simulink model "Mechanik_FensterSchlitten"  (R2021a)
settings: Solver=ode23s  StartTime=0.0  StopTime=10  MaxStep=1e-3  MinStep=1e-5  RelTol=1e-5  AbsTol=1e-5
values from neighbouring files (symbols this model uses):
  c = 10000    [Konstanten.m]
  d = 50    [Konstanten.m]
  da = 0.022    [Konstanten.m]
  eta = 0.7    [Konstanten.m]
  FR_Gleit = 4*mueG*FD    (= 27.5555)    [Konstanten.m]
  FR_Haft = (mF+mS)*g+0.1    (= 31.492)    [Konstanten.m]
  g = 9.81    [Konstanten.m]
  i = 1/49    (= 0.0204081632653)    [Konstanten.m]
  J = 1.8    [Konstanten.m]
  k3 = k4    (= 0.0315)    [Konstanten.m]
  k4 = M_Mot/Ia    (= 0.0315)    [Konstanten.m]
  ki = 100    [Konstanten.m]
  ki_U = 100    [Konstanten.m]
  kp = 100    [Konstanten.m]
  kp_U = 100    [Konstanten.m]
  L = Ta*Ra    (= 0.00161202272727)    [Konstanten.m]
  mF = 2.3    [Konstanten.m]
  mS = 0.9    [Konstanten.m]
  Ra = (Ua-UbN)/Ia    (= 1.81534090909)    [Konstanten.m]
settings Model: Creator=johannes  LastModifiedBy=johannes
settings SolverCC: ZeroCrossAlgorithm=Adaptive
settings DebuggingCC: IgnoredZcDiagnostic=none

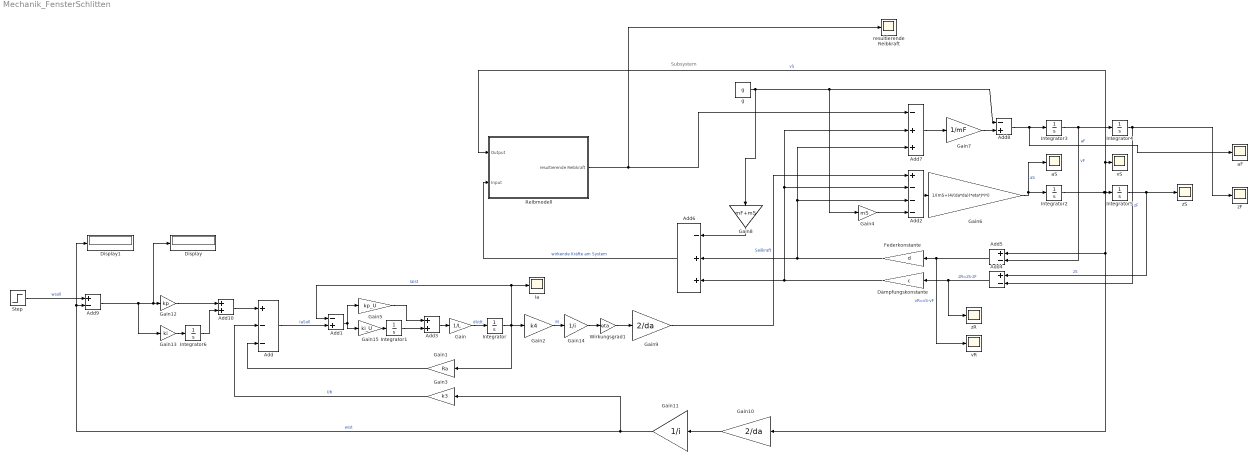
== system Mechanik_FensterSchlitten ==
  note: Subsystem
  Add : Sum  Inputs=+--
  Add1 : Sum  Inputs=-+
  Add10 : Sum
  Add2 : Sum  Inputs=+---
  Add3 : Sum
  Add4 : Sum  Inputs=+-
  Add5 : Sum  Inputs=+-
  Add6 : Sum  Inputs=-++
  Add7 : Sum  Inputs=-++
  Add8 : Sum  Inputs=-+
  Add9 : Sum  Inputs=+-
  Display : Display
  Display1 : Display
  Dämpfungskonstante : Gain  Gain=c
  Federkonstante : Gain  Gain=d
  Gain : Gain  Gain=1/L
  Gain1 : Gain  Gain=Ra
  Gain10 : Gain  Gain=2/da
  Gain11 : Gain  Gain=1/i
  Gain12 : Gain  Gain=kp
  Gain13 : Gain  Gain=ki
  Gain14 : Gain  Gain=1/i
  Gain15 : Gain  Gain=ki_U
  Gain2 : Gain  Gain=k4
  Gain3 : Gain  Gain=k3
  Gain4 : Gain  Gain=mS
  Gain5 : Gain  Gain=kp_U
  Gain6 : Gain  Gain=1/(mS+(4/(da*da))*eta*J*i*i)
  Gain7 : Gain  Gain=1/mF
  Gain8 : Gain  Gain=mF+mS
  Gain9 : Gain  Gain=2/da
  Ia : Scope
  Integrator{,1,3..6} (6 alike) : Integrator
  Integrator2 : Integrator  InitialCondition=1
  Reibmodell : Subsystem
  Step : Step  After=20  SampleTime=0
  Wirkungsgrad1 : Gain  Gain=eta
  aF : Scope
  aS : Scope
  g : Constant  Value=g
  resultierende Reibkraft : Scope
  vR : Scope
  vS : Scope
  zF : Scope
  zR : Scope
  zS : Scope
  wires:
  Gain9/1 -> Add2/1  "Seilkraft"
  Integrator/1 -> Add1/1, Ia/1, Gain2/1, Gain1/1  "IaIst"
  Gain3/1 -> Add/2  "Ub"
  Gain1/1 -> Add/3
  Gain/1 -> Integrator/1  "dI/dt"
  Dämpfungskonstante/1 -> Add6/3, Add7/2, Add2/2
  Federkonstante/1 -> Add6/2, Add7/3, Add2/3
  Gain8/1 -> Add6/1
  Add6/1 -> Reibmodell/2(Input)  "wirkende Kräfte am System"
  Integrator4/1 -> zF/1, Add4/2  "zF"
  Add2/1 -> Gain6/1
  Add7/1 -> Gain7/1
  Gain7/1 -> Add8/2
  Integrator3/1 -> Add5/2, Integrator4/1  "vF"
  Add8/1 -> aF/1, Integrator3/1  "aF"
  Integrator2/1 -> Gain10/1, Add5/1, Reibmodell/1(Output), vS/1, Integrator5/1  "vS"
  Gain6/1 -> Integrator2/1, aS/1  "aS"
  Reibmodell/1(resultierende Reibkraft) -> Add7/1, resultierende Reibkraft/1
  Add4/1 -> zR/1, Dämpfungskonstante/1  "zR=zS-zF"
  Add5/1 -> vR/1, Federkonstante/1  "vR=vS-vF"
  Integrator5/1 -> Add4/1, zS/1  "zS"
  g/1 -> Gain4/1, Add8/1, Gain8/1
  Gain10/1 -> Gain11/1
  Gain11/1 -> Gain3/1, Display1/1, Add9/2  "wist"
  Step/1 -> Add9/1  "wsoll"
  Add9/1 -> Display/1, Gain12/1, Gain13/1
  Gain13/1 -> Integrator6/1
  Add10/1 -> Add/1
  Integrator6/1 -> Add10/2
  Gain12/1 -> Add10/1
  Gain14/1 -> Wirkungsgrad1/1
  Gain2/1 -> Gain14/1  "M"
  Wirkungsgrad1/1 -> Gain9/1
  Gain4/1 -> Add2/4
  Add/1 -> Add1/2  "IaSoll"
  Integrator1/1 -> Add3/2
  Gain5/1 -> Add3/1
  Add1/1 -> Gain15/1, Gain5/1
  Gain15/1 -> Integrator1/1
  Add3/1 -> Gain/1

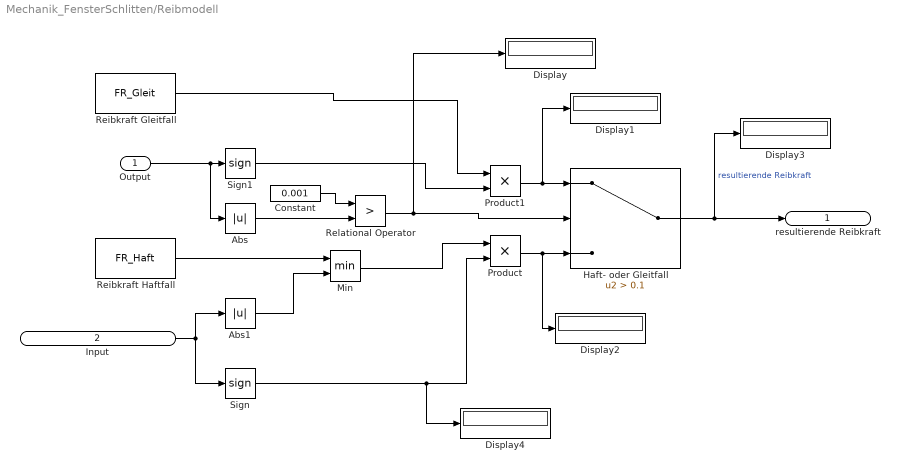
== system Mechanik_FensterSchlitten/Reibmodell ==
  Output : Inport
  Input : Inport  Port=2
  Abs : Abs
  Abs1 : Abs
  Constant : Constant  Value=0.001
  Display{,1..4} (5 alike) : Display
  Haft- oder Gleitfall : Switch  Criteria=u2 > Threshold  Threshold=0.1
  Min : MinMax  Inputs=2
  Product : Product
  Product1 : Product
  Reibkraft Gleitfall : Constant  Value=FR_Gleit
  Reibkraft Haftfall : Constant  Value=FR_Haft  VectorParams1D=off
  Relational Operator : RelationalOperator  Operator=>  OutDataTypeStr=boolean  RndMeth=Simplest
  Sign : Signum
  Sign1 : Signum
  resultierende Reibkraft : Outport
  wires:
  Haft- oder Gleitfall/1 -> Display3/1, resultierende Reibkraft/1  "resultierende Reibkraft"
  Product1/1 -> Display1/1, Haft- oder Gleitfall/1
  Output/1 -> Abs/1, Sign1/1
  Input/1 -> Sign/1, Abs1/1
  Min/1 -> Product/1
  Reibkraft Haftfall/1 -> Min/1
  Abs1/1 -> Min/2
  Product/1 -> Display2/1, Haft- oder Gleitfall/3
  Sign1/1 -> Product1/2
  Reibkraft Gleitfall/1 -> Product1/1
  Abs/1 -> Relational Operator/2
  Constant/1 -> Relational Operator/1
  Relational Operator/1 -> Display/1, Haft- oder Gleitfall/2
  Sign/1 -> Display4/1, Product/2
